simulink model "CLKinSim"  (R2012b)
settings: Solver=FixedStepDiscrete  StartTime=0.0  StopTime=1200  FixedStep=0.001  RelTol=1e-3
values from neighbouring files (symbols this model uses):
  baselineBias = [-0.1; -0.2]    [kinSim_buildWorkspace.m]    (also in runKinSim.m = opts.baselineBias(:))
  biasCorrectionEnable = false    [kinSim_buildWorkspace.m]    (also in runKinSim.m = true)
  biasCorrectionInitial = zeros(2,1)    [kinSim_buildWorkspace.m]    (also in runKinSim.m)
  biasCorrectionInitialMeans = zeros(4,1)    [kinSim_buildWorkspace.m]    (also in runKinSim.m)
  biasCorrectionMeansTau = double(1000*120)    [kinSim_buildWorkspace.m]    (also in runKinSim.m = double(opts.biasCorrectionMeansTau))
  biasCorrectionTau = double(1000*120)    [kinSim_buildWorkspace.m]    (also in runKinSim.m = double(opts.biasCorrectionTau))
  biasCorrectionType = uint16(0)    [kinSim_buildWorkspace.m]    (also in runKinSim.m = uint16(DecoderConstants.BIAS_CORRECTION_BEATA))
  biasCorrectionVelocityThreshold = double(0)    [kinSim_buildWorkspace.m]    (also in runKinSim.m = double(speedThreshold))
  cursorDiameter = double(30)    [kinSim_buildWorkspace.m]    (also in runKinSim.m)
  dwellTime = uint16(1000)    [kinSim_buildWorkspace.m]    (also in runKinSim.m = uint16(900))
  keyboard = uint16(keyboardConstants.KEYBOARD_GRID_6X6)    [kinSim_buildWorkspace.m]
  keyboardDims = uint16([screenMidPoint - [gridWidth gridHeight]/2 gridWidth gridHeight])    [kinSim_buildWorkspace.m]    (also in runKinSim.m)
  latency = uint16(100)    [kinSim_buildWorkspace.m]    (also in runKinSim.m = uint16(opts.latency))
  maxAccel = double(0.1)    [kinSim_buildWorkspace.m]    (also in runKinSim.m = double(0.005))
  maxVel = double(0.5)    [kinSim_buildWorkspace.m]    (also in runKinSim.m = double(1))
  numTrials = uint16(MAX_TRIALS)    [kinSim_buildWorkspace.m]    (also in runKinSim.m)
  runInRealTime = false    [kinSim_buildWorkspace.m]
  targetOrder = zeros([1 MAX_TRIALS],'uint16')    [kinSim_buildWorkspace.m]    (also in runKinSim.m = uint16(floor(rand(1,MAX_TRIALS)*36)+1))
  taskType = uint16(0)    [kinSim_buildWorkspace.m]    (also in runKinSim.m)
  trialTimeout = uint16(15000)    [kinSim_buildWorkspace.m]    (also in runKinSim.m = uint16(2500))
  vNoiseStd = double(0.1)    [kinSim_buildWorkspace.m]    (also in runKinSim.m = double(2))
  x = zeros(1,MAX_TRIALS,'uint16')    [runKinSim.m]
undefined symbols (not defined in the file or in its folder): dfilt, displayShape, displayShape_1, displayShape_10, displayShape_2, displayShape_3, displayShape_4, displayShape_5, displayShape_6, displayShape_7, displayShape_8, displayShape_9, fdesignblkfcn, gcbh, height, height_1, height_10, height_2, height_3, height_4, height_5, height_6, height_7, height_8, height_9, ID, ID_1, ID_10, ID_2, ID_3, ID_4, ID_5, ID_6, ID_7, ID_8, ID_9, numKeys, numKeys_1, numKeys_10, numKeys_2, numKeys_3, numKeys_4, numKeys_5, numKeys_6, numKeys_7, numKeys_8, numKeys_9, regionShape, regionShape_1, regionShape_10, regionShape_2, regionShape_3, regionShape_4, regionShape_5, regionShape_6, regionShape_7, regionShape_8, regionShape_9, text, text_1 ... (+74)
libraries: dspindex x3, dspmtrx3 x2, dspnetwork x2, simulink x1, commnoisgen2 x1, dsparch4 x1, realtime_pacer_lib x1
settings Model: SimulationMode=rapid-accelerator  ExtModeTrigDuration=100  Creator=Chethan  LastModifiedBy=Chethan
settings DataIOCC: SaveFinalState=on  SaveOutput=off  SaveState=on  StateSaveName=tmp_raccel_xout  TimeSaveName=tmp_raccel_tout
settings OptimizationCC: InlineParams=on  EnhancedBackFolding=on  RollThreshold=2  EfficientMapNaN2IntZero=off  SimCompilerOptimization=On
settings HardwareCC: TargetIntDivRoundTo=Zero  TargetEndianess=LittleEndian  TargetHWDeviceType=MATLAB Host  ProdEqTarget=off
settings RTWCC: SystemTargetFile=raccel.tlc  TemplateMakefile=raccel_default_tmf  RTWVerbose=off  ProcessScript=raccel_make_rtw_hook  RTWUseSimCustomCode=on
settings CodeAppCC: GenerateComments=off  MaxIdLength=128  MangleLength=10  SimulinkBlockComments=off
settings RaccelTargetCC: CodeReplacementLibrary=ANSI_C  ERTMultiwordTypeDef=System defined  ERTMultiwordLength=256  IsPILTarget=off  ParMdlRefBuildCompliant=off  GeneratePreprocessorConditionals=Disable all  ERTFirstTimeCompliant=off  MultiInstanceERTCode=off  EnableShiftOperators=on  ENABLE_SLEXEC_SSBRIDGE=off  RTWCAPISignals=off  RTWCAPIParams=off

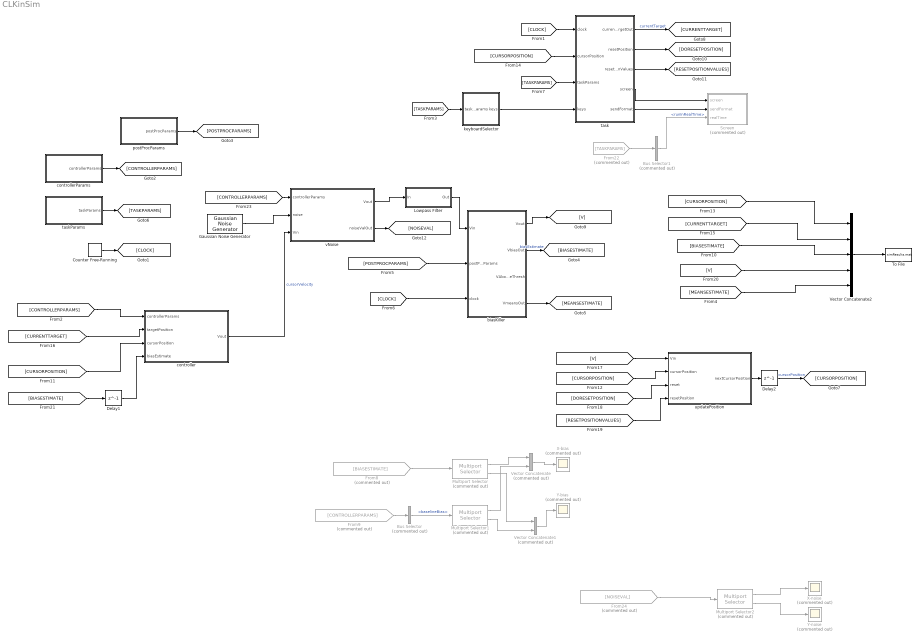
== system CLKinSim ==
  Bus Selector : BusSelector  Commented=on  OutputSignals=baselineBias
  Bus Selector1 : BusSelector  Commented=on  OutputSignals=runInRealTime
  Counter Free-Running : simulink/Sources/Counter Free-Running  NumBits=32  tsamp=-1
  Delay1 : Delay  DelayLength=1
  Delay2 : Delay  DelayLength=1
  From22 : From  Commented=on  GotoTag=TASKPARAMS
  From24 : From  Commented=on  GotoTag=NOISEVAL
  From8 : From  Commented=on  GotoTag=BIASESTIMATE
  From9 : From  Commented=on  GotoTag=CONTROLLERPARAMS
  Gaussian Noise Generator : commnoisgen2/Gaussian Noise Generator  m=[0;0]  d=[1;1]  s=41  Ts=0.001  frameBased=off  sampPerFrame=1  orient=off  outDataType=double
  Lowpass Filter : Subsystem  DialogController=fdesignblkfcn  InitFcn=fdesignblkfcn(gcbh, {'InitFcn'});  mask(Lowpass Filter){}
      mask help: Design a lowpass filter
      settings: CopyFcn=fdesignblkfcn(gcbh, {'CopyFcn'});
      mask Help: helpview(mapfilelocation('dsp'), 'dsplowpassfilter');
      mask Display: disp('Lowpass')
  Multiport Selector : dspindex/Multiport Selector  Commented=on  rowsOrCols=Rows  idxCellArray={ 1 2 }  idxErrMode=Clip Index
  Multiport Selector1 : dspindex/Multiport Selector  Commented=on  rowsOrCols=Rows  idxCellArray={ 1 2 }  idxErrMode=Clip Index
  Multiport Selector2 : dspindex/Multiport Selector  Commented=on  rowsOrCols=Rows  idxCellArray={ 1 2 }  idxErrMode=Clip Index
  Screen : Subsystem  Commented=on
  To File : ToFile  Filename=simResults.mat  MatrixName=results
  Vector Concatenate : Concatenate  Commented=on
  Vector Concatenate1 : Concatenate  Commented=on
  Vector Concatenate2 : Concatenate  NumInputs=5
  X-bias : Scope  Commented=on
      settings: TimeRange=200  YMin=-0.5  YMax=1.25
  X-noise : Scope  Commented=on
      settings: TimeRange=200  YMin=-4.5  YMax=3.5  SaveName=ScopeData3
  Y-bias : Scope  Commented=on
      settings: TimeRange=200  YMin=-0.025  YMax=0.025
  Y-noise : Scope  Commented=on
      settings: TimeRange=200  YMin=-0.1  YMax=0.9  SaveName=ScopeData2
  biasKiller : MATLAB Function  TreatAsAtomicUnit=on
  controller : MATLAB Function  TreatAsAtomicUnit=on
  controllerParams : Subsystem
  keyboardSelector : Subsystem
  postProcParams : Subsystem
  task : MATLAB Function  TreatAsAtomicUnit=on
  taskParams : Subsystem
  updatePosition : MATLAB Function  TreatAsAtomicUnit=on
  vNoise : MATLAB Function  TreatAsAtomicUnit=on
  wires:
  taskParams/1(taskParams) -> [TASKPARAMS]
  [TASKPARAMS] -> task/3(taskParams)
  Counter Free-Running/1 -> [CLOCK]
  [CLOCK] -> task/1(clock)
  updatePosition/1(nextCursorPosition) -> Delay2/1
  controllerParams/1(controllerParams) -> [CONTROLLERPARAMS]
  [CONTROLLERPARAMS] -> controller/1(controllerParams)
  task/4(screen) -> Screen/1(screen)
  task/5(sendFormat) -> Screen/2(sendFormat)
  keyboardSelector/1(keys) -> task/4(keys)
  [TASKPARAMS] -> keyboardSelector/1(taskParams)
  postProcParams/1(postProcParams) -> [POSTPROCPARAMS]
  [POSTPROCPARAMS] -> biasKiller/2(postProcParams)
  [CLOCK] -> biasKiller/3(clock)
  biasKiller/2(VbiasOut) -> [BIASESTIMATE]  "biasEstimate"
  biasKiller/4(VmeansOut) -> [MEANSESTIMATE]
  From9/1 -> Bus Selector/1
  From8/1 -> Multiport Selector/1
  Bus Selector/1 -> Multiport Selector1/1  "<baselineBias>"
  Multiport Selector/1 -> Vector Concatenate/1
  Multiport Selector1/1 -> Vector Concatenate/2
  Multiport Selector/2 -> Vector Concatenate1/1
  Multiport Selector1/2 -> Vector Concatenate1/2
  Vector Concatenate1/1 -> Y-bias/1
  Vector Concatenate/1 -> X-bias/1
  Vector Concatenate2/1 -> To File/1
  [BIASESTIMATE] -> Vector Concatenate2/3
  [CURSORPOSITION] -> controller/3(cursorPosition)
  [CURSORPOSITION] -> updatePosition/2(cursorPosition)
  [CURSORPOSITION] -> Vector Concatenate2/1
  [CURSORPOSITION] -> task/2(cursorPosition)
  Delay2/1 -> [CURSORPOSITION]  "cursorPosition"
  [CURRENTTARGET] -> Vector Concatenate2/2
  [CURRENTTARGET] -> controller/2(targetPosition)
  task/1(currentTargetOut) -> [CURRENTTARGET]  "currentTarget"
  [V] -> updatePosition/1(Vin)
  task/2(resetPosition) -> [DORESETPOSITION]
  task/3(resetPositionValues) -> [RESETPOSITIONVALUES]
  [DORESETPOSITION] -> updatePosition/3(reset)
  [RESETPOSITIONVALUES] -> updatePosition/4(resetPosition)
  [V] -> Vector Concatenate2/4
  [MEANSESTIMATE] -> Vector Concatenate2/5
  Delay1/1 -> controller/4(biasEstimate)
  [BIASESTIMATE] -> Delay1/1
  Bus Selector1/1 -> Screen/3(realTime)  "<runInRealTime>"
  biasKiller/1(Vout) -> [V]
  From22/1 -> Bus Selector1/1
  controller/1(Vout) -> vNoise/3(Vin)  "cursorVelocity"
  [CONTROLLERPARAMS] -> vNoise/1(controllerParams)
  Gaussian Noise Generator/1 -> vNoise/2(noise)
  Multiport Selector2/2 -> Y-noise/1
  vNoise/2(noiseValOut) -> [NOISEVAL]
  From24/1 -> Multiport Selector2/1
  Multiport Selector2/1 -> X-noise/1
  vNoise/1(Vout) -> Lowpass Filter/1(In)
  Lowpass Filter/1(Out) -> biasKiller/1(Vin)

== system CLKinSim/Lowpass Filter ==
  In : Inport
  Generated Filter Block : dsparch4/Biquad Filter  Tag=BlockMethodSubSystem  IIRFiltStruct=Direct form II  CoeffSource=Specify via dialog  BiQuadCoeffs=[0.25000004152994421 0.50000008305988841 0.25000004152994421 1 -1.9321316100426329 0.93436028275159677]  a0Flag=Warning  IC=0  ICnum=0  ICden=0  denAccumFracLength=30  denProdOutputFracLength=30  secondMemoryFracLength=15  roundingMode=Floor  overflowMode=off  ScaleValues=[0.0022286723387373755;1]  optimizeScaleValues=off  ScaleValueMode=Specify via input port (g)  scaleValueFracLength=14  FilterSource=Specify via dialog  dfiltObjectName=dfilt.df2tsos([1 0.3 0.4],[1 0.1 0.2])
  Out : Outport
  wires:
  In/1 -> Generated Filter Block/1
  Generated Filter Block/1 -> Out/1

== system CLKinSim/Screen ==
  screen : Inport  OutDataTypeStr=Bus: fileLoggerFormatAndData
  sendFormat : Inport  Port=2  OutDataTypeStr=boolean
  realTime : Inport  Port=3
  Bus Selector6 : BusSelector  OutputSignals=data.send,data.data,format.format
  Screen - Control : Subsystem
  Screen - Data : Subsystem
  run in real time : Subsystem  TreatAsAtomicUnit=on
  wires:
  Bus Selector6/2 -> Screen - Data/1(data)  "<data>"
  Bus Selector6/1 -> Screen - Data/Enable  "<send>"
  screen/1 -> Bus Selector6/1
  Bus Selector6/3 -> Screen - Control/1(data)  "<format>"
  sendFormat/1 -> Screen - Control/Enable
  realTime/1 -> run in real time/Enable

== system CLKinSim/controllerParams ==
  BusOutput : BusCreator  Inputs=maxVel,latency,vNoiseStd,maxAccel,baselineBias  OutDataTypeStr=Bus: controllerParams
  baselineBias : Constant  Value=baselineBias
  latency : Constant  Value=latency
  maxAccel : Constant  Value=maxAccel
  maxVel : Constant  Value=maxVel
  vNoiseStd : Constant  Value=vNoiseStd
  controllerParams : Outport
  wires:
  maxVel/1 -> BusOutput/1  "maxVel"
  latency/1 -> BusOutput/2  "latency"
  vNoiseStd/1 -> BusOutput/3  "vNoiseStd"
  maxAccel/1 -> BusOutput/4  "maxAccel"
  baselineBias/1 -> BusOutput/5  "baselineBias"
  BusOutput/1 -> controllerParams/1

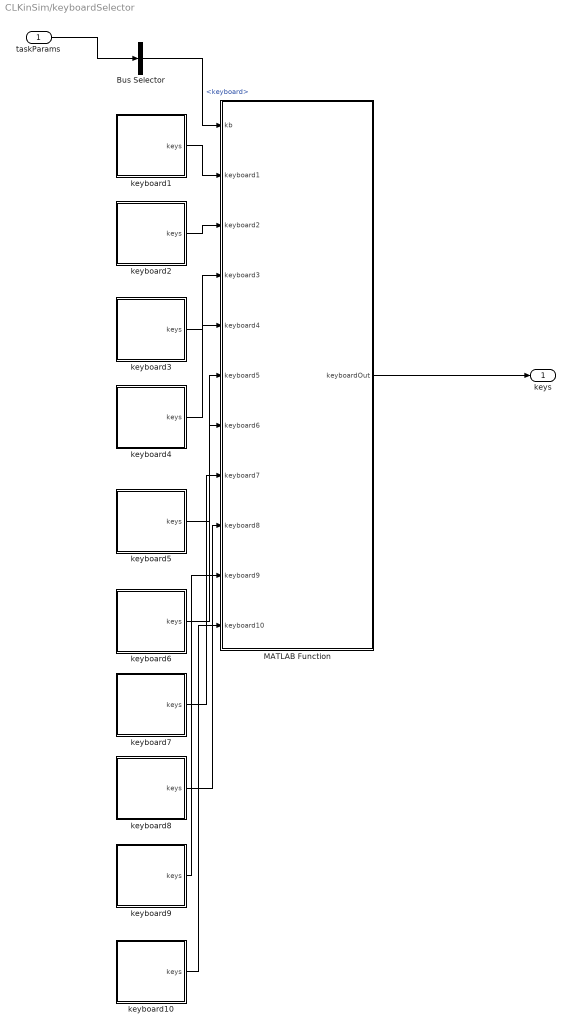
== system CLKinSim/keyboardSelector ==
  taskParams : Inport
  Bus Selector : BusSelector  OutputSignals=keyboard
  MATLAB Function : MATLAB Function  TreatAsAtomicUnit=on
  keyboard1 : Subsystem
  keyboard10 : Subsystem
  keyboard2 : Subsystem
  keyboard3 : Subsystem
  keyboard4 : Subsystem
  keyboard5 : Subsystem
  keyboard6 : Subsystem
  keyboard7 : Subsystem
  keyboard8 : Subsystem
  keyboard9 : Subsystem
  keys : Outport  OutDataTypeStr=Bus: keysParamsBus
  wires:
  keyboard1/1(keys) -> MATLAB Function/2(keyboard1)
  keyboard2/1(keys) -> MATLAB Function/3(keyboard2)
  MATLAB Function/1(keyboardOut) -> keys/1
  keyboard3/1(keys) -> MATLAB Function/4(keyboard3)
  keyboard4/1(keys) -> MATLAB Function/5(keyboard4)
  keyboard5/1(keys) -> MATLAB Function/6(keyboard5)
  keyboard6/1(keys) -> MATLAB Function/7(keyboard6)
  keyboard7/1(keys) -> MATLAB Function/8(keyboard7)
  keyboard8/1(keys) -> MATLAB Function/9(keyboard8)
  keyboard9/1(keys) -> MATLAB Function/10(keyboard9)
  keyboard10/1(keys) -> MATLAB Function/11(keyboard10)
  Bus Selector/1 -> MATLAB Function/1(kb)  "<keyboard>"
  taskParams/1 -> Bus Selector/1

== system CLKinSim/postProcParams ==
  BusOutput : BusCreator  Inputs=biasCorrectionVelocityThreshold,biasCorrectionTau,biasCorrectionEnable,biasCorrectionInitial,biasCorrectionType,biasCorrectionInitialMeans,biasCorrectionMeansTau  OutDataTypeStr=Bus: postProcParams
  biasCorrectionEnable : Constant  Value=biasCorrectionEnable
  biasCorrectionInitial : Constant  Value=biasCorrectionInitial
  biasCorrectionInitialMeans : Constant  Value=biasCorrectionInitialMeans
  biasCorrectionMeansTau : Constant  Value=biasCorrectionMeansTau
  biasCorrectionTau : Constant  Value=biasCorrectionTau
  biasCorrectionType : Constant  Value=biasCorrectionType
  biasCorrectionVelocityThreshold : Constant  Value=biasCorrectionVelocityThreshold
  postProcParams : Outport
  wires:
  biasCorrectionVelocityThreshold/1 -> BusOutput/1  "biasCorrectionVelocityThreshold"
  biasCorrectionTau/1 -> BusOutput/2  "biasCorrectionTau"
  biasCorrectionEnable/1 -> BusOutput/3  "biasCorrectionEnable"
  biasCorrectionInitial/1 -> BusOutput/4  "biasCorrectionInitial"
  biasCorrectionType/1 -> BusOutput/5  "biasCorrectionType"
  biasCorrectionInitialMeans/1 -> BusOutput/6  "biasCorrectionInitialMeans"
  biasCorrectionMeansTau/1 -> BusOutput/7  "biasCorrectionMeansTau"
  BusOutput/1 -> postProcParams/1

== system CLKinSim/taskParams ==
  BusOutput : BusCreator  Inputs=taskType,keyboard,keyboardDims,cursorDiameter,targetOrder,trialTimeout,numTrials,runInRealTime,dwellTime  OutDataTypeStr=Bus: taskParams
  cursorDiameter : Constant  Value=cursorDiameter
  dwellTime : Constant  Value=dwellTime
  keyboard : Constant  Value=keyboard
  keyboardDims : Constant  Value=keyboardDims
  numTrials : Constant  Value=numTrials
  runInRealTime : Constant  Value=runInRealTime
  targetOrder : Constant  Value=targetOrder
  taskType : Constant  Value=taskType
  trialTimeout : Constant  Value=trialTimeout
  taskParams : Outport
  wires:
  taskType/1 -> BusOutput/1  "taskType"
  keyboard/1 -> BusOutput/2  "keyboard"
  keyboardDims/1 -> BusOutput/3  "keyboardDims"
  cursorDiameter/1 -> BusOutput/4  "cursorDiameter"
  targetOrder/1 -> BusOutput/5  "targetOrder"
  trialTimeout/1 -> BusOutput/6  "trialTimeout"
  numTrials/1 -> BusOutput/7  "numTrials"
  runInRealTime/1 -> BusOutput/8  "runInRealTime"
  dwellTime/1 -> BusOutput/9  "dwellTime"
  BusOutput/1 -> taskParams/1

== system CLKinSim/Screen/Screen - Control ==
  data : Inport
  Enable : EnablePort
  MATLAB Function : MATLAB Function  TreatAsAtomicUnit=on
  Transpose : dspmtrx3/Transpose  Hermitian=off  overflowFlag=off
  UDP Send : dspnetwork/UDP Send  remoteURL='255.255.255.255'  remotePort=modelConstants.screen.CTRL_RECV_PORT  localURL='255.255.255.255'  localPortSource=Automatically determine  localPort=-1  sampletime=-1  blockPlatform=WINDOWS  separateLengthPort=0
  wires:
  data/1 -> MATLAB Function/1(u)
  MATLAB Function/1(y) -> Transpose/1
  Transpose/1 -> UDP Send/1

== system CLKinSim/Screen/Screen - Data ==
  data : Inport
  Enable : EnablePort
  MATLAB Function : MATLAB Function  TreatAsAtomicUnit=on
  Transpose : dspmtrx3/Transpose  Hermitian=off  overflowFlag=off
  UDP Send : dspnetwork/UDP Send  remoteURL='255.255.255.255'  remotePort=modelConstants.screen.DATA_RECV_PORT  localURL='255.255.255.255'  localPortSource=Automatically determine  localPort=-1  sampletime=-1  blockPlatform=WINDOWS  separateLengthPort=0
  wires:
  data/1 -> MATLAB Function/1(u)
  MATLAB Function/1(y) -> Transpose/1
  Transpose/1 -> UDP Send/1

== system CLKinSim/Screen/run in real time ==
  Enable : EnablePort
  Real-Time Pacer : realtime_pacer_lib/Real-Time Pacer  simTimePerRealTime=1

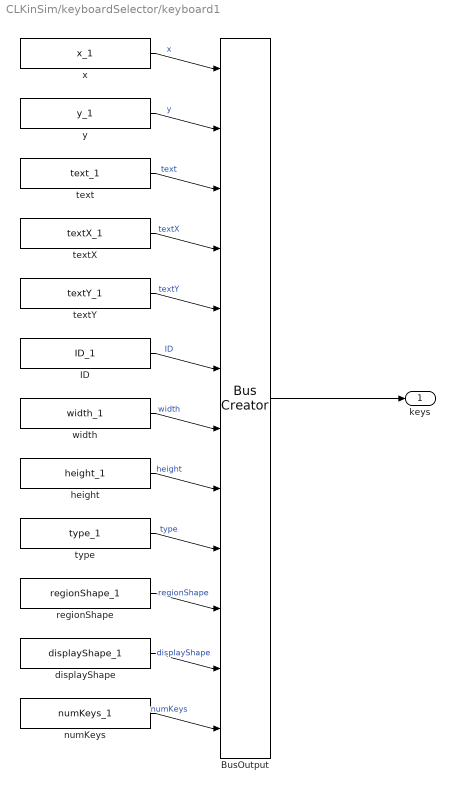
== system CLKinSim/keyboardSelector/keyboard1 ==
  BusOutput : BusCreator  Inputs=x,y,text,textX,textY,ID,width,height,type,regionShape,displayShape,numKeys  OutDataTypeStr=Bus: keysParamsBus
  ID : Constant  Value=ID_1
  displayShape : Constant  Value=displayShape_1
  height : Constant  Value=height_1
  numKeys : Constant  Value=numKeys_1
  regionShape : Constant  Value=regionShape_1
  text : Constant  Value=text_1
  textX : Constant  Value=textX_1
  textY : Constant  Value=textY_1
  type : Constant  Value=type_1
  width : Constant  Value=width_1
  x : Constant  Value=x_1
  y : Constant  Value=y_1
  keys : Outport
  wires:
  x/1 -> BusOutput/1  "x"
  y/1 -> BusOutput/2  "y"
  text/1 -> BusOutput/3  "text"
  textX/1 -> BusOutput/4  "textX"
  textY/1 -> BusOutput/5  "textY"
  ID/1 -> BusOutput/6  "ID"
  width/1 -> BusOutput/7  "width"
  height/1 -> BusOutput/8  "height"
  type/1 -> BusOutput/9  "type"
  regionShape/1 -> BusOutput/10  "regionShape"
  displayShape/1 -> BusOutput/11  "displayShape"
  numKeys/1 -> BusOutput/12  "numKeys"
  BusOutput/1 -> keys/1

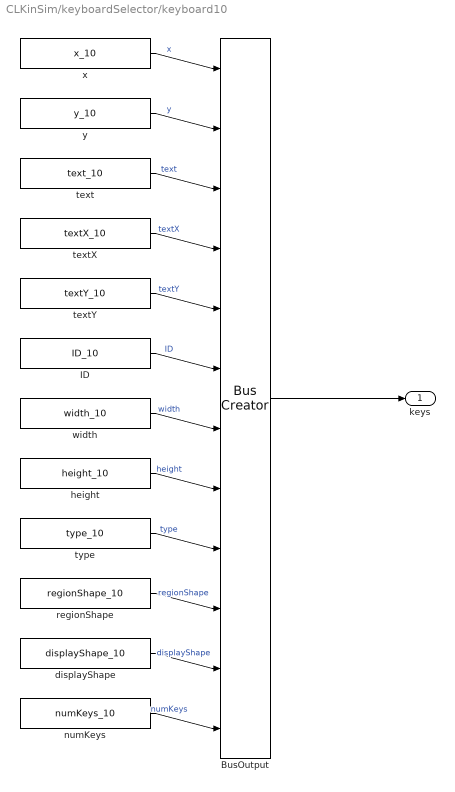
== system CLKinSim/keyboardSelector/keyboard10 ==
  BusOutput : BusCreator  Inputs=x,y,text,textX,textY,ID,width,height,type,regionShape,displayShape,numKeys  OutDataTypeStr=Bus: keysParamsBus
  ID : Constant  Value=ID_10
  displayShape : Constant  Value=displayShape_10
  height : Constant  Value=height_10
  numKeys : Constant  Value=numKeys_10
  regionShape : Constant  Value=regionShape_10
  text : Constant  Value=text_10
  textX : Constant  Value=textX_10
  textY : Constant  Value=textY_10
  type : Constant  Value=type_10
  width : Constant  Value=width_10
  x : Constant  Value=x_10
  y : Constant  Value=y_10
  keys : Outport  OutDataTypeStr=Bus: keysParamsBus
  wires:
  x/1 -> BusOutput/1  "x"
  y/1 -> BusOutput/2  "y"
  text/1 -> BusOutput/3  "text"
  textX/1 -> BusOutput/4  "textX"
  textY/1 -> BusOutput/5  "textY"
  ID/1 -> BusOutput/6  "ID"
  width/1 -> BusOutput/7  "width"
  height/1 -> BusOutput/8  "height"
  type/1 -> BusOutput/9  "type"
  regionShape/1 -> BusOutput/10  "regionShape"
  displayShape/1 -> BusOutput/11  "displayShape"
  numKeys/1 -> BusOutput/12  "numKeys"
  BusOutput/1 -> keys/1

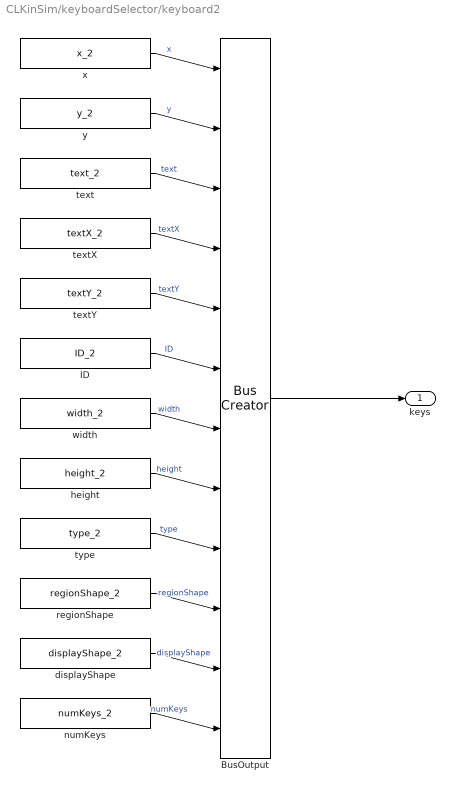
== system CLKinSim/keyboardSelector/keyboard2 ==
  BusOutput : BusCreator  Inputs=x,y,text,textX,textY,ID,width,height,type,regionShape,displayShape,numKeys  OutDataTypeStr=Bus: keysParamsBus
  ID : Constant  Value=ID_2
  displayShape : Constant  Value=displayShape_2
  height : Constant  Value=height_2
  numKeys : Constant  Value=numKeys_2
  regionShape : Constant  Value=regionShape_2
  text : Constant  Value=text_2
  textX : Constant  Value=textX_2
  textY : Constant  Value=textY_2
  type : Constant  Value=type_2
  width : Constant  Value=width_2
  x : Constant  Value=x_2
  y : Constant  Value=y_2
  keys : Outport  OutDataTypeStr=Bus: keysParamsBus
  wires:
  x/1 -> BusOutput/1  "x"
  y/1 -> BusOutput/2  "y"
  text/1 -> BusOutput/3  "text"
  textX/1 -> BusOutput/4  "textX"
  textY/1 -> BusOutput/5  "textY"
  ID/1 -> BusOutput/6  "ID"
  width/1 -> BusOutput/7  "width"
  height/1 -> BusOutput/8  "height"
  type/1 -> BusOutput/9  "type"
  regionShape/1 -> BusOutput/10  "regionShape"
  displayShape/1 -> BusOutput/11  "displayShape"
  numKeys/1 -> BusOutput/12  "numKeys"
  BusOutput/1 -> keys/1

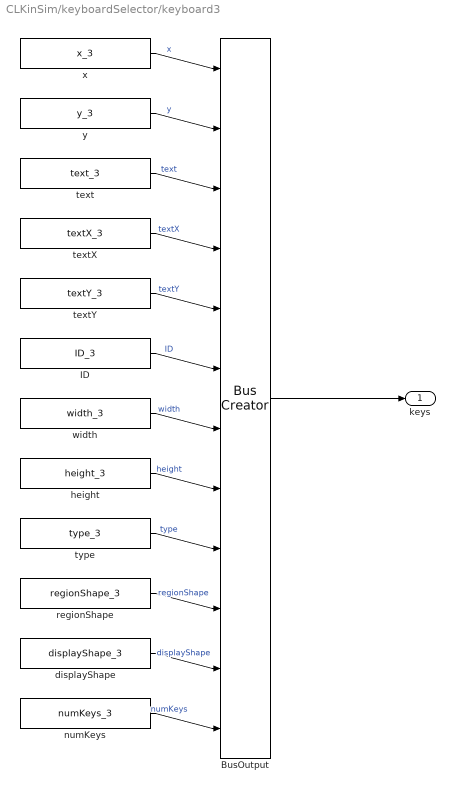
== system CLKinSim/keyboardSelector/keyboard3 ==
  BusOutput : BusCreator  Inputs=x,y,text,textX,textY,ID,width,height,type,regionShape,displayShape,numKeys  OutDataTypeStr=Bus: keysParamsBus
  ID : Constant  Value=ID_3
  displayShape : Constant  Value=displayShape_3
  height : Constant  Value=height_3
  numKeys : Constant  Value=numKeys_3
  regionShape : Constant  Value=regionShape_3
  text : Constant  Value=text_3
  textX : Constant  Value=textX_3
  textY : Constant  Value=textY_3
  type : Constant  Value=type_3
  width : Constant  Value=width_3
  x : Constant  Value=x_3
  y : Constant  Value=y_3
  keys : Outport  OutDataTypeStr=Bus: keysParamsBus
  wires:
  x/1 -> BusOutput/1  "x"
  y/1 -> BusOutput/2  "y"
  text/1 -> BusOutput/3  "text"
  textX/1 -> BusOutput/4  "textX"
  textY/1 -> BusOutput/5  "textY"
  ID/1 -> BusOutput/6  "ID"
  width/1 -> BusOutput/7  "width"
  height/1 -> BusOutput/8  "height"
  type/1 -> BusOutput/9  "type"
  regionShape/1 -> BusOutput/10  "regionShape"
  displayShape/1 -> BusOutput/11  "displayShape"
  numKeys/1 -> BusOutput/12  "numKeys"
  BusOutput/1 -> keys/1

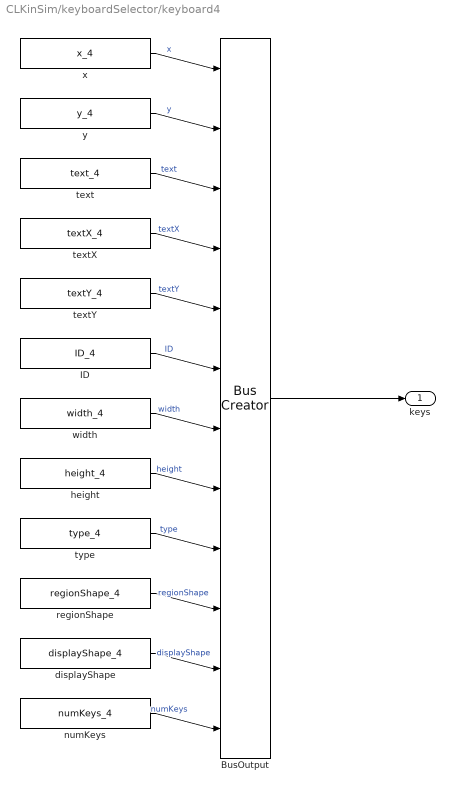
== system CLKinSim/keyboardSelector/keyboard4 ==
  BusOutput : BusCreator  Inputs=x,y,text,textX,textY,ID,width,height,type,regionShape,displayShape,numKeys  OutDataTypeStr=Bus: keysParamsBus
  ID : Constant  Value=ID_4
  displayShape : Constant  Value=displayShape_4
  height : Constant  Value=height_4
  numKeys : Constant  Value=numKeys_4
  regionShape : Constant  Value=regionShape_4
  text : Constant  Value=text_4
  textX : Constant  Value=textX_4
  textY : Constant  Value=textY_4
  type : Constant  Value=type_4
  width : Constant  Value=width_4
  x : Constant  Value=x_4
  y : Constant  Value=y_4
  keys : Outport  OutDataTypeStr=Bus: keysParamsBus
  wires:
  x/1 -> BusOutput/1  "x"
  y/1 -> BusOutput/2  "y"
  text/1 -> BusOutput/3  "text"
  textX/1 -> BusOutput/4  "textX"
  textY/1 -> BusOutput/5  "textY"
  ID/1 -> BusOutput/6  "ID"
  width/1 -> BusOutput/7  "width"
  height/1 -> BusOutput/8  "height"
  type/1 -> BusOutput/9  "type"
  regionShape/1 -> BusOutput/10  "regionShape"
  displayShape/1 -> BusOutput/11  "displayShape"
  numKeys/1 -> BusOutput/12  "numKeys"
  BusOutput/1 -> keys/1

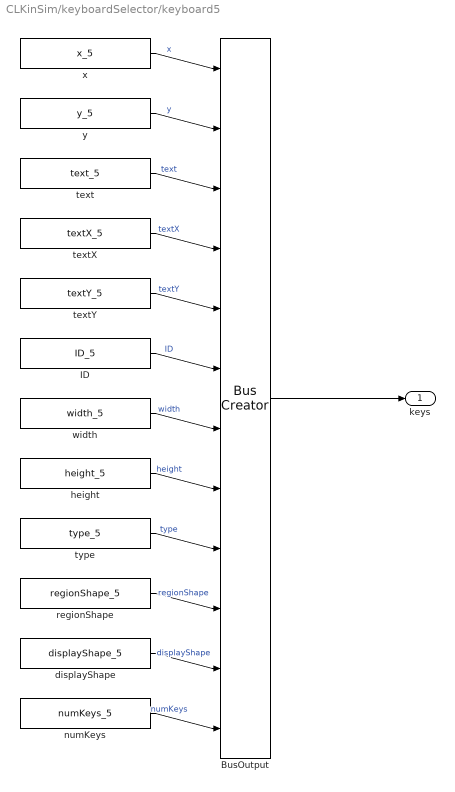
== system CLKinSim/keyboardSelector/keyboard5 ==
  BusOutput : BusCreator  Inputs=x,y,text,textX,textY,ID,width,height,type,regionShape,displayShape,numKeys  OutDataTypeStr=Bus: keysParamsBus
  ID : Constant  Value=ID_5
  displayShape : Constant  Value=displayShape_5
  height : Constant  Value=height_5
  numKeys : Constant  Value=numKeys_5
  regionShape : Constant  Value=regionShape_5
  text : Constant  Value=text_5
  textX : Constant  Value=textX_5
  textY : Constant  Value=textY_5
  type : Constant  Value=type_5
  width : Constant  Value=width_5
  x : Constant  Value=x_5
  y : Constant  Value=y_5
  keys : Outport  OutDataTypeStr=Bus: keysParamsBus
  wires:
  x/1 -> BusOutput/1  "x"
  y/1 -> BusOutput/2  "y"
  text/1 -> BusOutput/3  "text"
  textX/1 -> BusOutput/4  "textX"
  textY/1 -> BusOutput/5  "textY"
  ID/1 -> BusOutput/6  "ID"
  width/1 -> BusOutput/7  "width"
  height/1 -> BusOutput/8  "height"
  type/1 -> BusOutput/9  "type"
  regionShape/1 -> BusOutput/10  "regionShape"
  displayShape/1 -> BusOutput/11  "displayShape"
  numKeys/1 -> BusOutput/12  "numKeys"
  BusOutput/1 -> keys/1

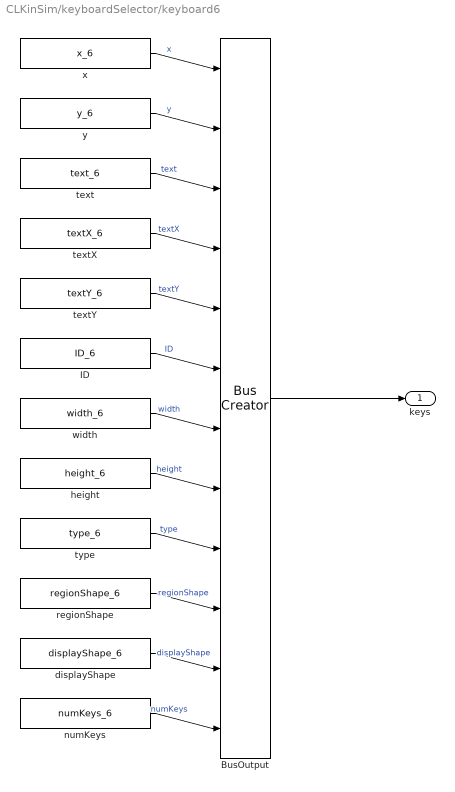
== system CLKinSim/keyboardSelector/keyboard6 ==
  BusOutput : BusCreator  Inputs=x,y,text,textX,textY,ID,width,height,type,regionShape,displayShape,numKeys  OutDataTypeStr=Bus: keysParamsBus
  ID : Constant  Value=ID_6
  displayShape : Constant  Value=displayShape_6
  height : Constant  Value=height_6
  numKeys : Constant  Value=numKeys_6
  regionShape : Constant  Value=regionShape_6
  text : Constant  Value=text_6
  textX : Constant  Value=textX_6
  textY : Constant  Value=textY_6
  type : Constant  Value=type_6
  width : Constant  Value=width_6
  x : Constant  Value=x_6
  y : Constant  Value=y_6
  keys : Outport  OutDataTypeStr=Bus: keysParamsBus
  wires:
  x/1 -> BusOutput/1  "x"
  y/1 -> BusOutput/2  "y"
  text/1 -> BusOutput/3  "text"
  textX/1 -> BusOutput/4  "textX"
  textY/1 -> BusOutput/5  "textY"
  ID/1 -> BusOutput/6  "ID"
  width/1 -> BusOutput/7  "width"
  height/1 -> BusOutput/8  "height"
  type/1 -> BusOutput/9  "type"
  regionShape/1 -> BusOutput/10  "regionShape"
  displayShape/1 -> BusOutput/11  "displayShape"
  numKeys/1 -> BusOutput/12  "numKeys"
  BusOutput/1 -> keys/1

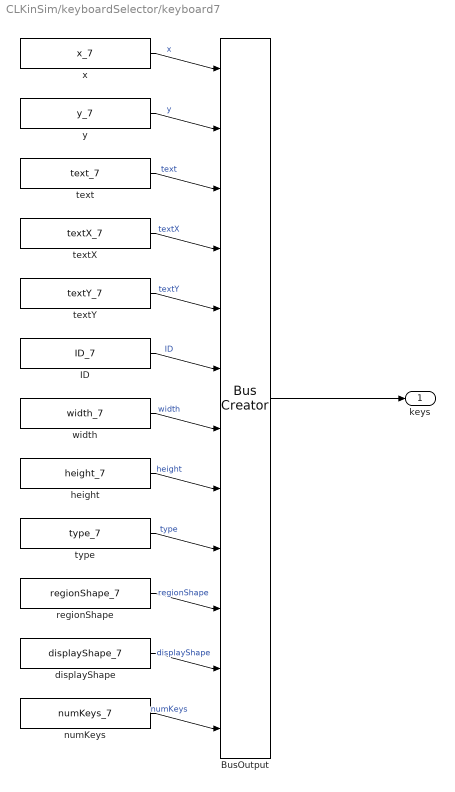
== system CLKinSim/keyboardSelector/keyboard7 ==
  BusOutput : BusCreator  Inputs=x,y,text,textX,textY,ID,width,height,type,regionShape,displayShape,numKeys  OutDataTypeStr=Bus: keysParamsBus
  ID : Constant  Value=ID_7
  displayShape : Constant  Value=displayShape_7
  height : Constant  Value=height_7
  numKeys : Constant  Value=numKeys_7
  regionShape : Constant  Value=regionShape_7
  text : Constant  Value=text_7
  textX : Constant  Value=textX_7
  textY : Constant  Value=textY_7
  type : Constant  Value=type_7
  width : Constant  Value=width_7
  x : Constant  Value=x_7
  y : Constant  Value=y_7
  keys : Outport  OutDataTypeStr=Bus: keysParamsBus
  wires:
  x/1 -> BusOutput/1  "x"
  y/1 -> BusOutput/2  "y"
  text/1 -> BusOutput/3  "text"
  textX/1 -> BusOutput/4  "textX"
  textY/1 -> BusOutput/5  "textY"
  ID/1 -> BusOutput/6  "ID"
  width/1 -> BusOutput/7  "width"
  height/1 -> BusOutput/8  "height"
  type/1 -> BusOutput/9  "type"
  regionShape/1 -> BusOutput/10  "regionShape"
  displayShape/1 -> BusOutput/11  "displayShape"
  numKeys/1 -> BusOutput/12  "numKeys"
  BusOutput/1 -> keys/1

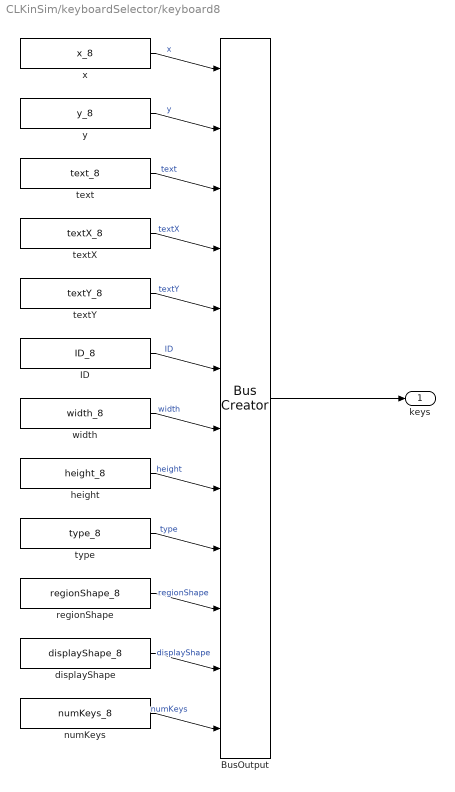
== system CLKinSim/keyboardSelector/keyboard8 ==
  BusOutput : BusCreator  Inputs=x,y,text,textX,textY,ID,width,height,type,regionShape,displayShape,numKeys  OutDataTypeStr=Bus: keysParamsBus
  ID : Constant  Value=ID_8
  displayShape : Constant  Value=displayShape_8
  height : Constant  Value=height_8
  numKeys : Constant  Value=numKeys_8
  regionShape : Constant  Value=regionShape_8
  text : Constant  Value=text_8
  textX : Constant  Value=textX_8
  textY : Constant  Value=textY_8
  type : Constant  Value=type_8
  width : Constant  Value=width_8
  x : Constant  Value=x_8
  y : Constant  Value=y_8
  keys : Outport  OutDataTypeStr=Bus: keysParamsBus
  wires:
  x/1 -> BusOutput/1  "x"
  y/1 -> BusOutput/2  "y"
  text/1 -> BusOutput/3  "text"
  textX/1 -> BusOutput/4  "textX"
  textY/1 -> BusOutput/5  "textY"
  ID/1 -> BusOutput/6  "ID"
  width/1 -> BusOutput/7  "width"
  height/1 -> BusOutput/8  "height"
  type/1 -> BusOutput/9  "type"
  regionShape/1 -> BusOutput/10  "regionShape"
  displayShape/1 -> BusOutput/11  "displayShape"
  numKeys/1 -> BusOutput/12  "numKeys"
  BusOutput/1 -> keys/1

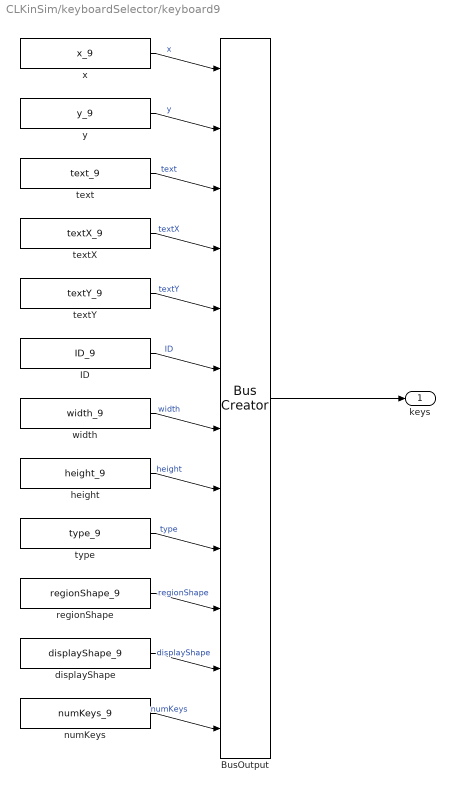
== system CLKinSim/keyboardSelector/keyboard9 ==
  BusOutput : BusCreator  Inputs=x,y,text,textX,textY,ID,width,height,type,regionShape,displayShape,numKeys  OutDataTypeStr=Bus: keysParamsBus
  ID : Constant  Value=ID_9
  displayShape : Constant  Value=displayShape_9
  height : Constant  Value=height_9
  numKeys : Constant  Value=numKeys_9
  regionShape : Constant  Value=regionShape_9
  text : Constant  Value=text_9
  textX : Constant  Value=textX_9
  textY : Constant  Value=textY_9
  type : Constant  Value=type_9
  width : Constant  Value=width_9
  x : Constant  Value=x_9
  y : Constant  Value=y_9
  keys : Outport  OutDataTypeStr=Bus: keysParamsBus
  wires:
  x/1 -> BusOutput/1  "x"
  y/1 -> BusOutput/2  "y"
  text/1 -> BusOutput/3  "text"
  textX/1 -> BusOutput/4  "textX"
  textY/1 -> BusOutput/5  "textY"
  ID/1 -> BusOutput/6  "ID"
  width/1 -> BusOutput/7  "width"
  height/1 -> BusOutput/8  "height"
  type/1 -> BusOutput/9  "type"
  regionShape/1 -> BusOutput/10  "regionShape"
  displayShape/1 -> BusOutput/11  "displayShape"
  numKeys/1 -> BusOutput/12  "numKeys"
  BusOutput/1 -> keys/1

== matlab function CLKinSim/updatePosition ==
  data: Vin input; nextCursorPosition output; cursorPosition input double size=[2 1]; reset input; resetPosition input double size=[2 1]
function nextCursorPosition  = updatePosition(Vin, cursorPosition, reset, resetPosition)

nextCursorPosition = cursorPosition + Vin;

if reset
    nextCursorPosition = resetPosition;
end

== matlab function CLKinSim/controller ==
  data: controllerParams input; targetPosition input; Vout output; cursorPosition input; biasEstimate input size=[2 1]
function Vout  = controller(controllerParams, targetPosition, cursorPosition, biasEstimate)

%controllerType = 'hoffarbib';
controllerType = 'constantaccel';

MAX_LATENCY = 1000;
% how long should a reach take, in MS?
reachTimeMS = double(500);

persistent V;
persistent lastPositions;
maxVel = controllerParams.maxVel;
maxAccel = controllerParams.maxAccel;
latency = controllerParams.latency;

persistent lastA;
persistent lastV;

if isempty(V)
    V=zeros([2,1]);
    lastPositions=zeros([2, MAX_LATENCY]);
    lastTargetPosition = double([0;0]);
    
    lastV=[0;0];
    lastA=[0;0];
end
A = zeros(2,1);
J = zeros(2,1);

% store the previous positions in case latency is used
lastPositions(:,1:latency-1) = lastPositions(:,2:latency);
lastPositions(:,latency) = cursorPosition;
lastX = lastPositions(:,1);


vToTarg = (double(targetPosition) - double(lastX));
nV = sqrt(sum(vToTarg.^2));

Vout=[0;0;];

if nV > 0 % only update V if we are not on target
    
    switch lower(controllerType)
        case 'hoffarbib'
            D = reachTimeMS;
            for ndim = 1:2
                q = double([lastX(ndim); lastV(ndim); lastA(ndim)]);
                qdot =   [0 1 0; ...
                          0 0 1; ...
                         -60/(D^3) -36/(D^2) -9/D] * q ...
                         + [0; 0; 60/(D^3)] * targetPosition(ndim);
                J(ndim) = qdot(3);
                A(ndim) = J(ndim) + lastA(ndim);
                V(ndim) = A(ndim) + lastV(ndim);
            end
            lastA = A;
            lastV = V;
            
            Vout = V + controllerParams.baselineBias;
            
        case 'constantaccel'
            unitToTarg = vToTarg ./nV;
            if nV * 0.01 > maxVel
                maxToTarg = unitToTarg * maxVel;
                desiredV = maxToTarg;
            else
                desiredV = vToTarg * 0.01;
            end
            Vdiff = desiredV - V;
            VdiffNorm = sqrt(sum(Vdiff.^2));
            if VdiffNorm <= maxAccel
                V = desiredV;
            else
                V = V + maxAccel * (Vdiff ./ VdiffNorm);
            end
            Vout = V + controllerParams.baselineBias;
        otherwise
            error('huh?');
    end
end

== matlab function CLKinSim/Screen/Screen - Control/MATLAB Function ==
  data: u input; y output
function y = padData(u)

z = uint8(zeros(1434, 1))';

z(1:length(u)) = u;

y = z';

== matlab function CLKinSim/vNoise ==
  data: controllerParams input; noise input; Vin input; Vout output; noiseValOut output
function [Vout,noiseValOut] = vNoise(controllerParams, noise, Vin)

persistent noiseVal;

if isempty(noiseVal)
    noiseVal = [0;0];
end

%noiseVal(2) = noiseVal(2) + noise(2) * controllerParams.vNoiseStd;

Vout = Vin + noise * controllerParams.vNoiseStd;
noiseValOut = noise * controllerParams.vNoiseStd;

== matlab function CLKinSim/Screen/Screen - Data/MATLAB Function ==
  data: u input; y output
function y = padData(u)

z = uint8(zeros(1434, 1))';

z(1:length(u)) = u;

y = z';

== matlab function CLKinSim/biasKiller ==
  data: Vout output; Vin input; postProcParams input; VbiasOut output; VAboveThresh output; VmeansOut output; clock input
function [Vout, VbiasOut, VAboveThresh, VmeansOut] = biasKiller(Vin, postProcParams, clock)

useFrankMod = true;

speedThreshold = postProcParams.biasCorrectionVelocityThreshold;
tau = postProcParams.biasCorrectionTau;
enable = postProcParams.biasCorrectionEnable;
biasCorrectionInitial = postProcParams.biasCorrectionInitial;
biasCorrectionType = postProcParams.biasCorrectionType;
biasCorrectionInitialMeans = postProcParams.biasCorrectionInitialMeans;
meansTau = postProcParams.biasCorrectionMeansTau;

persistent Vbias;
persistent VmeansXY;
persistent numPoints;
if isempty(Vbias)
    Vbias = zeros(size(Vin));
    VmeansXY = zeros([4 1]);
    numPoints = zeros([4 1])+40000;
end

if clock<100
    switch biasCorrectionType
        %% for the CP/PN bias killer, we are tracking 4 params (X- mean, X+ mean, Y- mean, Y+ mean)
        case DecoderConstants.BIAS_CORRECTION_CPPN
            VmeansXY = biasCorrectionInitialMeans;
            Vbias = biasCorrectionInitial;
        %% for Frank's unbiased killer, we are tracking 2 params (X bias, Y bias)
        case {DecoderConstants.BIAS_CORRECTION_FRANK, DecoderConstants.BIAS_CORRECTION_BEATA}
            Vbias = biasCorrectionInitial;
    end
end

VAboveThresh = false;

if enable && clock>100
    switch biasCorrectionType
        %% CP/PN Bias killer, 2014-12-11
        case DecoderConstants.BIAS_CORRECTION_CPPN
            velUnbiased = double(Vin) - double(Vbias);
            
            %% first handle X, then Y
            if norm(velUnbiased) > speedThreshold
                for dirInd = 1:2
                    meansTauCurrent = meansTau;
                    if velUnbiased(dirInd) < 0
                        velInd = 1+2*(dirInd-1);
                    else
                        velInd = 2+2*(dirInd-1);
                    end
                    %% adjust the X mean velocity for this direction
                    if isnan(VmeansXY(velInd))
                        VmeansXY(velInd) = velUnbiased(dirInd);
                        numPoints(velInd) = 1;
                    else
                        %if numPoints(velInd) < meansTau
                        %    numPoints(velInd) = numPoints(velInd)+1;
                        %    meansTauCurrent = numPoints(velInd);
                        %end
                        if useFrankMod
                            VmeansXY(velInd) = VmeansXY(velInd) + (velUnbiased(dirInd)-VmeansXY(velInd)) .* abs(velUnbiased(dirInd)-VmeansXY(velInd)) ./ double(meansTauCurrent);
                        else
                            VmeansXY(velInd) = VmeansXY(velInd) + (velUnbiased(dirInd)-VmeansXY(velInd))  ./ double(meansTauCurrent);
                        end
                    end
                end
                
                deltaMeansX = abs(VmeansXY(2))-abs(VmeansXY(1));
                deltaMeansY = abs(VmeansXY(4))-abs(VmeansXY(3));
                
                if ~isnan(deltaMeansX)
                    Vbias(1) = Vbias(1) + deltaMeansX ./ double(tau);
                end
                if ~isnan(deltaMeansY)
                    Vbias(2) = Vbias(2) + deltaMeansY ./ double(tau);
                end
                
            end
%            % correct the means estimates by the change in bias estimate
%            VmeansXY(1:2) = VmeansXY(1:2) - deltaMeansX ./ double(tau) ./ 2;
%            VmeansXY(3:4) = VmeansXY(3:4) - deltaMeansY ./ double(tau) ./ 2;
            
            
            %% Frank's unbiased killer
        case DecoderConstants.BIAS_CORRECTION_FRANK
            %% criteria for counting Vin towards Vbias:
            %%    speed must be greater than some threshold.
            
            speed = sqrt(sum((double(Vin)-double(Vbias)).^2));
            if (double(speed) > double(speedThreshold))
                Vbias = Vbias + (double(Vin)-Vbias).*(abs(double(Vin)-Vbias))./double(tau);
                VAboveThresh = true;
            end
        case DecoderConstants.BIAS_CORRECTION_BEATA
            %% criteria for counting Vin towards Vbias:
            %%    speed must be greater than some threshold.
            
            speed = sqrt(sum((double(Vin)-double(Vbias)).^2));
            if (double(speed) > double(speedThreshold))
                Vbias = Vbias + (double(Vin)-Vbias)./double(tau);
                VAboveThresh = true;
            end
    end
    Vout = double(Vin) - Vbias;
else
    Vout = double(Vin);
end

VbiasOut = Vbias;
VmeansOut = VmeansXY;

== matlab function CLKinSim/keyboardSelector/MATLAB Function ==
  data: kb input; keyboardOut output Bus: keysParamsBus; keyboard1 input Bus: keysParamsBus; keyboard2 input Bus: keysParamsBus; keyboard3 input; keyboard4 input; keyboard5 input; keyboard6 input; keyboard7 input; keyboard8 input; keyboard9 input; keyboard10 input
function keyboardOut = chooseKeyboard(kb, keyboard1, keyboard2, keyboard3, keyboard4, keyboard5, keyboard6, keyboard7, keyboard8, keyboard9, keyboard10)
%#codegen

k = uint16(kb);

switch k
    case uint16(keyboardConstants.KEYBOARD_QWERTY1)
        keyboardOut = keyboard1;
        
    case uint16(keyboardConstants.KEYBOARD_QWERTY2)
        keyboardOut = keyboard2;
        
    case uint16(keyboardConstants.KEYBOARD_GRID_6X6)
        keyboardOut = keyboard3;
        
    case uint16(keyboardConstants.KEYBOARD_GRID_7X7)
        keyboardOut = keyboard4;
        
    case uint16(keyboardConstants.KEYBOARD_GRID_8X8)
        keyboardOut = keyboard5;
        
    case uint16(keyboardConstants.KEYBOARD_GRID_9X9)
        keyboardOut = keyboard6;

    case uint16(keyboardConstants.KEYBOARD_GRID_10X10)
        keyboardOut = keyboard7;
    
    case uint16(keyboardConstants.KEYBOARD_QABCD)
        keyboardOut = keyboard8;

    case uint16(keyboardConstants.KEYBOARD_OPTIII)
        keyboardOut = keyboard9;

    case uint16(keyboardConstants.KEYBOARD_GRID_5X5)
        keyboardOut = keyboard10;
        
    otherwise
        keyboardOut = keyboard1;
end

== matlab function CLKinSim/task ==
  data: clock input; cursorPosition input; currentTargetOut output; taskParams input Bus: taskParams; resetPosition output; resetPositionValues output; screen output Bus: fileLoggerFormatAndData; sendFormat output; keys input
function [currentTargetOut,resetPosition, resetPositionValues, screen, sendFormat] = task(clock, cursorPosition, taskParams, keys)

TASK_NAME = 'CLKINSIM';
VERSION_ID = single(0.1);


persistent currentTarget taskState trialNum stateTimer holdTimer cumulativeDwell;
if isempty(currentTarget)
    currentTarget = uint16(0);
    taskState = uint16(0);
    trialNum = uint16(0);
    stateTimer = uint16(0);
	cumulativeDwell = initCumulativeDwell();
end

resetPosition = false;
resetPositionValues = [0;0];

keyboardDims = taskParams.keyboardDims;% uint16([240 90 1000 1000]);

overTarget = uint16(0);
cuedTarget = uint16(0);
overCuedTarget = uint16(0);

screenMidPoint = [960; 540];
cpshift = cursorPosition(1:2)+screenMidPoint;


if taskState ~= 0
    overTarget = isCursorOverTarget(keys, cpshift, keyboardDims,...
        false, false);
end

if trialNum
    currentTarget = taskParams.targetOrder(trialNum);
else
    currentTarget = uint16(0);
end

acquiredTarget = 0;
nextTarget = false;
switch taskState
    case uint16(0) %% waiting for task to start
        if clock >= 100
            taskState = uint16(1);
            stateTimer = uint16(0);
            trialNum = uint16(1);
            cumulativeDwell = initCumulativeDwell();
        end
    case uint16(1) %% running
        stateTimer = stateTimer+uint16(1);
        if overTarget
            cumulativeDwell(overTarget) = cumulativeDwell(overTarget) + uint16(1);
        end
        
        if overTarget && cumulativeDwell(overTarget) > taskParams.dwellTime
            acquiredTarget = overTarget;
            nextTarget = true;
        elseif taskParams.dwellTime && stateTimer>taskParams.trialTimeout
            nextTarget = true;
        end
        
        if nextTarget
            stateTimer = uint16(0);
            trialNum = trialNum + uint16(1);
            cumulativeDwell = initCumulativeDwell();
        end    
end


cuedTarget = currentTarget;

if currentTarget
    currentTargetPosXY = [keys.x(currentTarget)+keys.width(currentTarget)/2; keys.y(currentTarget)+keys.height(currentTarget)/2];
    currentTargetPos = keyboardToScreenCoords(currentTargetPosXY,keyboardDims) - screenMidPoint;
else
    currentTargetPos = [0;0];
end
sendFormat = false;
sendData = false;
if clock > 1 && clock < 100
    if mod(clock,10) == 0
        sendFormat = true;
    end
    
    resetPosition = true;
end

if clock >= 100 && mod(clock,10)==0
    sendData = true;
end


%% INITIALIZE TASK OUTPUT
fileLoggerData.data = uint8(zeros(1,1400));
fileLoggerData.dataLen = uint16(0);
fileLoggerData.fileName = uint8(zeros(1,20));
fileLoggerData.send = false;

fileLoggerFormat.format = uint8(zeros(1,1400));
fileLoggerFormat.formatLen = uint16(0);
fileLoggerFormat.fileName = uint8(zeros(1,20));

fileLoggerFormatAndData.format = fileLoggerFormat;
fileLoggerFormatAndData.data = fileLoggerData;

screen = fileLoggerFormatAndData;

currentTargetOut = currentTargetPos;
taskStateOut = taskState;


%% SEND DATA OUT TO VIZ
screen = packFileLoggerFormatAndData('screen', ...
    TASK_NAME, VERSION_ID, ...
    'clock', clock,...
    'state',taskStateOut,...
    'keyboard',uint16(keyboardConstants.KEYBOARD_GRID_6X6),...
    'keyboardDims',keyboardDims,...
    'numKeys',keys.numKeys(1),...
    'cursorPosition',cpshift,...
    'cursorDiameter',taskParams.cursorDiameter,...
    'cuedTarget', cuedTarget,...
    'overTarget', overTarget,...
    'overCuedTarget',overCuedTarget,...
    'taskType', taskParams.taskType...
    );

screen.data.send = sendData;

end

function x = initCumulativeDwell()
    x = zeros([1 uint16(100)],'uint16');
end
